simulink model "fullbridgeinverter1"  (R2021a)
settings: Solver=VariableStepAuto  StartTime=0.0  StopTime=100  RelTol=1e-3
libraries: spsIGBTDiodeLib x4, spsCurrentMeasurementLib x1, spsDCVoltageSourceLib x1, spsGroundLib x1, spsMultimeterLib x1, spsSeriesRLCBranchLib x1, spsVoltageMeasurementLib x1, spspowerguiLib x1
settings Model: Creator=User  LastModifiedBy=User

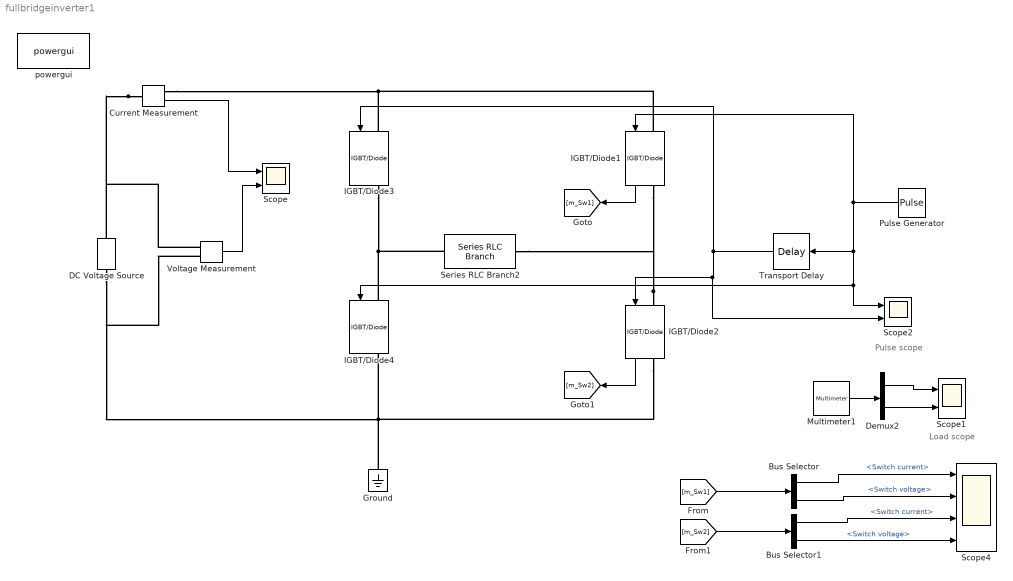
== system fullbridgeinverter1 ==
  note: Load scope
  note: Pulse scope
  Bus Selector : BusSelector  OutputSignals=Switch current,Switch voltage
  Bus Selector1 : BusSelector  OutputSignals=Switch current,Switch voltage
  Current Measurement : spsCurrentMeasurementLib/Current Measurement  PhasorSimulation=off  OutputType=Complex  PSBequivalent=0
  DC Voltage Source : spsDCVoltageSourceLib/DC Voltage Source  Amplitude=200  Measurements=None
  Demux2 : Demux  Outputs=2
  Ground : spsGroundLib/Ground  LConnTagsString=a
  IGBT/Diode{1..4} (4 alike) : spsIGBTDiodeLib/IGBT//Diode  Ron=1e-3  Rs=1e5  Cs=inf  Measurements=on
  Multimeter1 : spsMultimeterLib/Multimeter  PhasorSimulation=off  OutputType=Complex  sel=[1 2]  L=2  Gain=[1 1]  yselected={'Ub: Series RLC Branch2','Ib: Series RLC Branch2'};  PSBOutputType=1  PSBequivalent=0  AxesSetting=[0,0.1,-100,100]  Display=0  SavedBlockNames=-11
  Pulse Generator : DiscretePulseGenerator  PulseType=Time based  Period=0.02  PulseWidth=49.99
  Scope : Scope  NumInputPorts=2
  Scope1 : Scope  NumInputPorts=2
  Scope2 : Scope  NumInputPorts=2
  Scope4 : Scope  NumInputPorts=4
  Series RLC Branch2 : spsSeriesRLCBranchLib/Series RLC Branch  LConnTagsString=__new0  RConnTagsString=__new0  BranchType=RL  Resistance=100  Inductance=1  SetiL0=off  InitialCurrent=0  Capacitance=1e-6  Setx0=off  InitialVoltage=0  Measurements=Branch voltage and current
  Transport Delay : TransportDelay  DelayTime=0.01
  Voltage Measurement : spsVoltageMeasurementLib/Voltage Measurement  PhasorSimulation=off  OutputType=Complex  PSBequivalent=0
  powergui : spspowerguiLib/powergui  Priority=1  SimulationMode=Continuous  SampleTime=50e-6  frequency=60  Iterations=50  frequencyindice=0  Pbase=100e6  ErrMax=1e-4  UnitsV=kV  UnitsW=MW  buscounter=0  FunctionMessages=off  echomessages=off  EnableUseOfTLC=off  CurrentSourceSwitches=off  DisableSnubberDevices=off  DisableRonSwitches=off  DisableVfSwitches=off  DisplayEquations=off  AutomaticDiscreteSolvers=off  SolverType=Tustin/Backward Euler (TBE)  Interpol=off  ExternalGateDelay=off  methode=off  Ts=100  x0status=blocks  SPID=on  SwTol=0  HookPort=off  NonlinearTolerance=1e-4  nMaxIteration=100  ContinueOnMaxIteration=off  RestoreLinks=warning  ResistiveCurrentMeasurement=off  Frange=[0:2:500]  Ylog=off  Xlog=on  ShowGrid=off  save=off  variable=ZData  structure=0  ZoomFFT=off  StartTime=0.0  cycles=1  DisplayStyle=1  fundamental=60  FreqAxis=off  MaxFrequency=1000  frequencyindicesteady=1  RmsSteady=1  display=off
  wires:
  Bus Selector1/2 -> Scope4/4  "<Switch voltage>"
  Bus Selector1/1 -> Scope4/3  "<Switch current>"
  Bus Selector/1 -> Scope4/1  "<Switch current>"
  Bus Selector/2 -> Scope4/2  "<Switch voltage>"
  Transport Delay/1 -> IGBT/Diode3/1, Scope2/2, IGBT/Diode2/1
  [m_Sw2] -> Bus Selector1/1
  Pulse Generator/1 -> IGBT/Diode1/1, IGBT/Diode4/1, Scope2/1, Transport Delay/1
  Demux2/1 -> Scope1/1
  Current Measurement/1 -> Scope/1
  [m_Sw1] -> Bus Selector/1
  Multimeter1/1 -> Demux2/1
  Voltage Measurement/1 -> Scope/2
  IGBT/Diode2/1 -> [m_Sw2]
  Demux2/2 -> Scope1/2
  IGBT/Diode1/1 -> [m_Sw1]
  connections:
  IGBT/Diode2/LConn1 -- IGBT/Diode1/RConn1 -- Series RLC Branch2/RConn1
  Ground/LConn1 -- IGBT/Diode4/RConn1 -- DC Voltage Source/LConn1 -- Voltage Measurement/LConn2 -- IGBT/Diode2/RConn1
  Series RLC Branch2/LConn1 -- IGBT/Diode4/LConn1 -- IGBT/Diode3/RConn1
  IGBT/Diode1/LConn1 -- IGBT/Diode3/LConn1 -- Current Measurement/RConn1
  Current Measurement/LConn1 -- DC Voltage Source/RConn1 -- Voltage Measurement/LConn1
